simulink model "lab2_part1_model"  (R2023a)
settings: Solver=ode45  StartTime=0.0  StopTime=3  RelTol=1e-3
values from neighbouring files (symbols this model uses):
  A = [-6 -25 ... (first row only)    [lab2_part1.m]
  B = [25; 0]    [lab2_part1.m]
  C = eye(2)    [lab2_part1.m]
  D = [0; 0]    [lab2_part1.m]
settings Model: Creator=Jiadong_Hong  LastModifiedBy=Jiadong_Hong

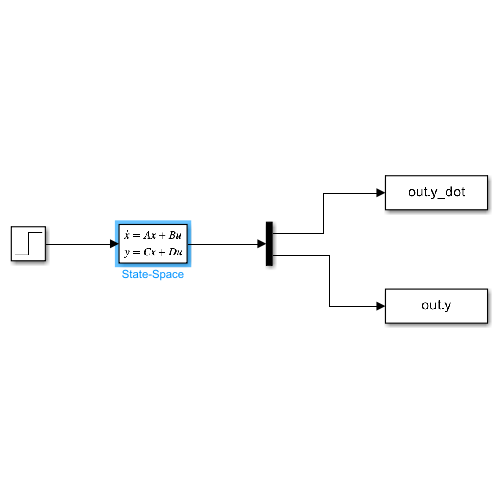
[thumbnail: Simulink's stored preview of the top-level diagram]
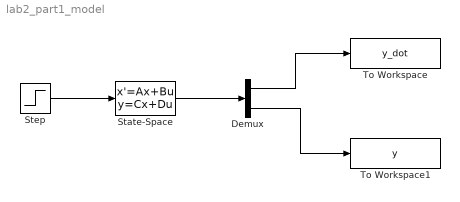
== system lab2_part1_model ==
  Demux : Demux  Outputs=2
  State-Space : StateSpace  A=A  B=B  C=C  D=D  InitialCondition=0
  Step : Step  Time=0  SampleTime=0
  To Workspace : ToWorkspace  VariableName=y_dot  SampleTime=-1
  To Workspace1 : ToWorkspace  VariableName=y  SampleTime=-1
  wires:
  Step/1 -> State-Space/1
  State-Space/1 -> Demux/1
  Demux/1 -> To Workspace/1
  Demux/2 -> To Workspace1/1
